simulink model "ex1"  (R2023b)
settings: Solver=FixedStepAuto  StartTime=0.0  StopTime=50  FixedStep=0.001  RelTol=1e-3
libraries: simulink_extras x4
settings Model: Creator=Andrei  LastModifiedBy=Andrei

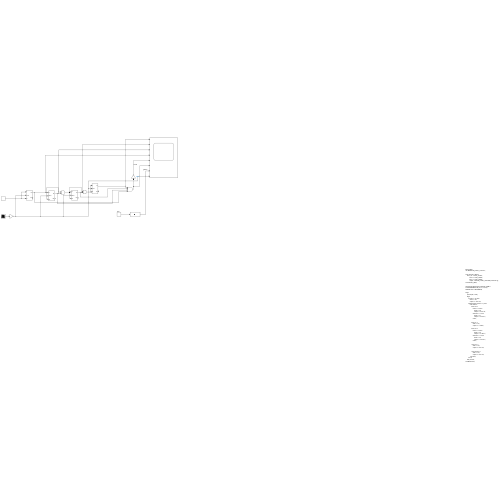
[thumbnail: Simulink's stored preview of the top-level diagram]
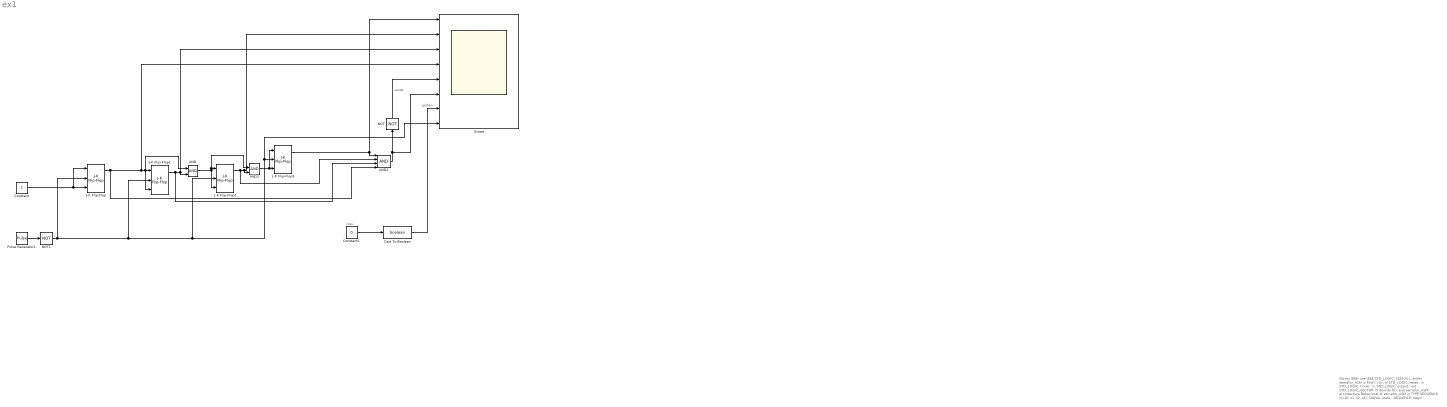
== system ex1 ==
  note: galben
  note: verde
  note: rosu
  note: library IEEE;
      | use IEEE.STD_LOGIC_1164.ALL;
      |
      | entity semafor_ASM is
      |     Port ( clk : in STD_LOGIC;
      |            reset : in STD_LOGIC;
      |            timer : in STD_LOGIC;
      |            output : out STD_LOGIC_VECTOR (5 downto 0));
      | end semafor_ASM;
      |
      | architecture Behavioral of semafor_ASM is
      | TYPE SEQUENCE IS (s0, s1, s2, s3);
      | SIGNAL state : SEQUENCE;
      |
      | begin
      |     process(clk, reset)
      |     begin
      |         if (reset <= '0') then
      |             state <= s0;
      |             output <= "011110";
      |         elsif(clk'event and clk = '1') then
      |             case state is
      |                 when s0 =>
      |                     if timer = '0' then
      |                         state <= s0;
      |                         output <= "011110";
      |                     elsif timer = '1' then
      |                         state <= s1;
      |                         output <= "011101";
      |                     end if;
      |
      |                 when s1 =>
      |                     state <= s2;
      |                     output <= "110011";
      |
      |                 when s2 =>
      |                     if timer = '0' then
      |                         state <= s2;
      |                         output <= "110011";
      |                     elsif timer = '1' then
      |                         state <= s3;
      |                         output <= "101011";
      |                     end if;
      |
      |                  when s3 =>
      |                     state <= s0;
      |                     output <= "011110";
      |
      |                  when others =>
      |                     state <= s0;
      |                     output <= "011110";
      |              end case;
      |         end if;
      |     end process;
      | end Behavioral;
  AND : Logic  IconShape=distinctive  AllPortsSameDT=off  OutDataTypeStr=boolean
  AND1 : Logic  IconShape=distinctive  AllPortsSameDT=off  OutDataTypeStr=boolean
  AND2 : Logic  Inputs=4  IconShape=distinctive  AllPortsSameDT=off  OutDataTypeStr=boolean
  Cast To Boolean : DataTypeConversion  OutDataTypeStr=boolean  SaturateOnIntegerOverflow=off  RndMeth=Floor
  Constant : Constant  OutDataTypeStr=boolean
  Constant1 : Constant  Value=0
  J-K Flip-Flop{,1..3} (4 alike) : simulink_extras/Flip Flops/J-K Flip-Flop  initial_condition=0
  NOT : Logic  Operator=NOT  IconShape=distinctive  AllPortsSameDT=off  OutDataTypeStr=boolean
  NOT1 : Logic  Operator=NOT  IconShape=distinctive  AllPortsSameDT=off  OutDataTypeStr=boolean
  Pulse Generator1 : DiscretePulseGenerator  PulseType=Time based  PulseWidth=5
  Scope : Scope  NumInputPorts=8
  wires:
  J-K Flip-Flop3/1 -> Scope/1, AND2/1
  J-K Flip-Flop1/1 -> AND2/3, Scope/3, AND/2
  J-K Flip-Flop2/1 -> AND2/2, Scope/2, AND1/2
  J-K Flip-Flop/1 -> AND2/4, Scope/4, J-K Flip-Flop1/3, AND/1, J-K Flip-Flop1/1
  AND/1 -> J-K Flip-Flop2/3, J-K Flip-Flop2/1, AND1/1
  AND1/1 -> J-K Flip-Flop3/1, J-K Flip-Flop3/3
  Constant/1 -> J-K Flip-Flop/1, J-K Flip-Flop/3
  Pulse Generator1/1 -> NOT1/1
  AND2/1 -> Scope/6, NOT/1
  Constant1/1 -> Cast To Boolean/1
  Cast To Boolean/1 -> Scope/7
  NOT/1 -> Scope/5
  NOT1/1 -> Scope/8, J-K Flip-Flop3/2, J-K Flip-Flop2/2, J-K Flip-Flop1/2, J-K Flip-Flop/2
